simulink model "Model_2a_H2_batteries_primary_clean"  (R2019a)
settings: Solver=FixedStepAuto  StartTime=0.0  StopTime=8760  FixedStep=1  RelTol=1e-3
libraries: simulink x7
settings Model: Creator=senja  LastModifiedBy=senja

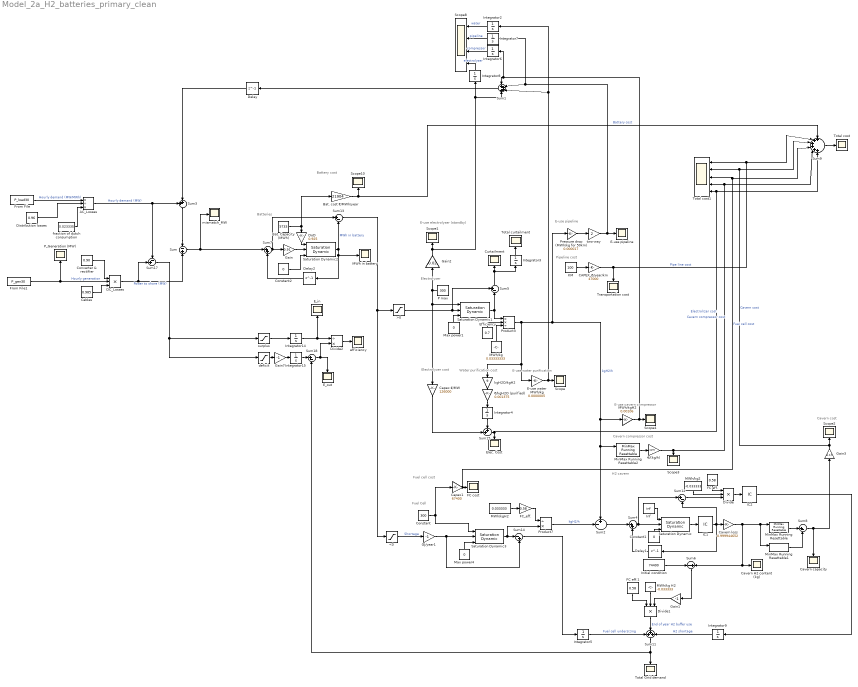
== system Model_2a_H2_batteries_primary_clean ==
  note: Water purification cost
  note: Batteries
  note: E-use pipeline
  note: E-use cavern compressor
  note: Cavern compressor cost
  note: Cavern cost
  note: E-use electrolyser (standby)
  note: E-use water purification
  note: Fuel cell cost
  note: Pipeline cost
  note: H2 cavern
  note: Fuel Cell
  note: Electrolyser
  note: Electrolyzer cost
  note: Battery cost
  <0 : Saturate  UpperLimit=0  LowerLimit=-inf
  >0 : Saturate  UpperLimit=inf  LowerLimit=-0
  AC_Losses : Product  Inputs=*/*
  Bat. Capacity (MWh) : Constant  Value=5733
  Bat. cost €/MWh/year : Gain  Gain=21904
  CAPEX_€/year/km : Gain  Gain=47000
  Cables : Constant  Value=0.985
  Capex €/MW : Gain  Gain=126000
  Capex1 : Gain  Gain=67400
  "Cavern H2 content (kg) " : Scope
  Cavern capacity : Scope
  Cavern loss : Gain  Gain=0.999944652
  Constant : Constant  Value=300
  Constant1 : Constant  Value=0
  Constant2 : Constant  Value=0
  Converter & rectifier : Constant  Value=0.90
  Curtailment : Scope
  DC_Losses : Product  Inputs=3
  Delay : Delay  DelayLength=1  InitialCondition=0
  Delay1 : Delay  DelayLength=1  InitialCondition=0
  Delay2 : Delay  DelayLength=1
  Distribution losses : Constant  Value=0.96
  Divide : Product  Inputs=***
  Divide1 : Product  Inputs=***
  Divide2 : Product  Inputs=/*
  DoD : Gain  Gain=0.925
  E-use pipeline : Scope
  E-use water MWh/kg : Gain  Gain=0.0000005
  E_in : Scope
  E_out : Scope
  Efficiency : Constant  Value=0.7
  Elec. Cost : Scope
  FC cost : Scope
  FC eff. : Constant  Value=0.58
  FC eff.1 : Constant  Value=0.58
  FC_eff. : Gain  Gain=0.58
  From File : FromFile  FileName=P_load30  SampleTime=0
  From File1 : FromFile  FileName=P_gen30  SampleTime=0
  GJ/year1 : Gain  Gain=-1
  Gain : Gain  Gain=0.91
  Gain1 : Gain  Gain=-1
  Gain2 : Gain  Gain=0.02
  Gain3 : Gain  Gain=0.17
  Gain7 : Gain  Gain=-1
  IC1 : InitialCondition  Value=74400
  IC2 : InitialCondition  Value=0
  Inf : Constant  Value=inf  OutDataTypeStr=Inherit: Inherit via back propagation
  Initial condition : Constant  Value=74400
  Integrator{2..9,14..15} (10 alike) : Integrator
  KM : Constant  Value=100
  "MWh in battery " : Scope
  MWh/kg : Constant  Value=0.03333333
  MWh/kg H2 : Constant  Value=-0.033333
  MWh/kg2 : Constant  Value=-0.033333
  MWh/kgH2 : Constant  Value=0.033333
  "MWh/kgH2 " : Gain  Gain=0.00106
  Max power1 : Constant  Value=0
  Max power4 : Constant  Value=0
  MinMax Running Resettable : simulink/Math Operations/MinMax Running Resettable  Function=max  vinit=0.0
  MinMax Running Resettable1 : simulink/Math Operations/MinMax Running Resettable  Function=min  vinit=0.0
  MinMax Running Resettable2 : simulink/Math Operations/MinMax Running Resettable  Function=max  vinit=0.0
  P max : Constant  Value=300
  P_Generation (MW) : Scope
  Pressure drop (MWh/kg for 50km) : Gain  Gain=0.000017
  Product3 : Product  Inputs=**/
  Product7 : Product  Inputs=/*
  Saturation Dynamic : simulink/Discontinuities/Saturation Dynamic  OutMin=0  OutMax=[]  OutDataTypeStr=Inherit: Same as second input  OutDataType=fixdt(1, 16)  OutScaling=2^-10  DoSatur=off
  Saturation Dynamic1 : simulink/Discontinuities/Saturation Dynamic  OutMin=[]  OutMax=[]  OutDataTypeStr=Inherit: Same as second input  OutDataType=fixdt(1, 16)  OutScaling=2^-10  DoSatur=off
  Saturation Dynamic2 : simulink/Discontinuities/Saturation Dynamic  OutMin=[]  OutMax=[]  OutDataTypeStr=Inherit: Same as second input  OutDataType=fixdt(1, 16)  OutScaling=2^-10  DoSatur=off
  Saturation Dynamic3 : simulink/Discontinuities/Saturation Dynamic  OutMin=[]  OutMax=[]  OutDataTypeStr=Inherit: Same as second input  OutDataType=fixdt(1, 16)  OutScaling=2^-10  DoSatur=off
  Scope{,1..4,10} (6 alike) : Scope
  Scope8 : Scope  NumInputPorts=4
  Sum : Sum  Inputs=-|+
  Sum1 : Sum  Inputs=++++
  Sum11 : Sum  Inputs=+++
  Sum{8,12..13,18} (4 alike) : Sum  Inputs=|+-
  Sum14 : Sum  Inputs=|-+
  Sum15 : Sum  Inputs=++|
  Sum17 : Sum  Inputs=-+|
  Sum2 : Sum  Inputs=+-|
  Sum3 : Sum  Inputs=++|
  Sum4 : Sum  Inputs=|++
  Sum5 : Sum  Inputs=+-|
  Sum6 : Sum  Inputs=-|+
  Sum7 : Sum  Inputs=|++
  Sum9 : Sum  Inputs=++++++
  Total Grid demand : Scope
  Total cost : Scope
  Total cost1 : Scope  NumInputPorts=5
  Total curtailment : Scope
  Transportation cost : Scope
  deficit : Saturate  UpperLimit=0  LowerLimit=-inf
  efficiency : Scope
  fraction of dutch consumption : Constant  Value=0.023335
  kgH2O/kgH2 : Gain  Gain=9
  mismatch_MW : Scope
  surplus : Saturate  UpperLimit=inf  LowerLimit=0
  two-way : Gain  Gain=2
  €/(kg/h) : Gain  Gain=1170
  €/kgH2O (purified) : Gain  Gain=0.001375
  wires:
  From File/1 -> AC_Losses/1  "Hourly demand (MW/MWh)"
  Efficiency/1 -> Product3/2
  fraction of dutch consumption/1 -> AC_Losses/3
  Distribution losses/1 -> AC_Losses/2
  Cables/1 -> DC_Losses/3
  Converter & rectifier/1 -> DC_Losses/1
  DC_Losses/1 -> Sum17/2, Sum/2  "Power to shore (MW)"
  >0/1 -> Sum5/1, Saturation Dynamic1/2
  <0/1 -> GJ/year1/1  "Shortage"
  AC_Losses/1 -> Sum3/1, Sum17/1  "Hourly demand (MW)"
  From File1/1 -> P_Generation (MW)/1, DC_Losses/2  "Hourly generation"
  Max power1/1 -> Saturation Dynamic1/3
  Saturation Dynamic1/1 -> Sum5/2, Product3/1
  Capex €/MW/1 -> Sum15/2
  Sum15/1 -> Elec. Cost/1, Sum9/6, Total cost1/5  "Electrolizer cost"
  €/kgH2O (purified)/1 -> Integrator4/1
  P max/1 -> Saturation Dynamic1/1, Capex €/MW/1, Gain2/1
  GJ/year1/1 -> Sum14/2, Saturation Dynamic3/2
  KM/1 -> CAPEX_€/year/km/1
  CAPEX_€/year/km/1 -> Total cost1/1, Sum9/2, Transportation cost/1  "Pipe line cost"
  Product3/1 -> E-use water MWh/kg/1, kgH2O/kgH2/1, "MWh/kgH2 "/1, MinMax Running Resettable2/1, Sum2/1, Pressure drop (MWh/kg for 50km)/1  "kgH2/h"
  Sum/1 -> Sum7/1, mismatch_MW/1
  Sum9/1 -> Total cost/1
  Constant/1 -> Saturation Dynamic3/1, Capex1/1
  Max power4/1 -> Saturation Dynamic3/3
  Saturation Dynamic3/1 -> Sum14/1, Product7/2
  MWh/kgH2/1 -> FC_eff./1
  Integrator3/1 -> Total curtailment/1
  kgH2O/kgH2/1 -> €/kgH2O (purified)/1
  Integrator4/1 -> Sum15/1
  MWh/kg/1 -> Product3/3
  Capex1/1 -> Total cost1/3, Sum9/4, FC cost/1  "Fuel cell cost"
  FC_eff./1 -> Product7/1
  Product7/1 -> Sum2/2  "kgH2/h"
  MinMax Running Resettable/1 -> Sum8/1
  MinMax Running Resettable1/1 -> Sum8/2
  Sum8/1 -> Cavern capacity/1, Gain3/1
  Sum5/1 -> Integrator3/1, Curtailment/1
  FC eff./1 -> Divide/1
  MWh/kg2/1 -> Divide/2
  Divide/1 -> IC2/1
  Sum14/1 -> Integrator5/1
  Initial condition/1 -> Sum6/1
  Integrator5/1 -> Sum11/1  "Fuel cell undersizing"
  Sum6/1 -> Gain1/1
  Sum11/1 -> Sum18/2, Total Grid demand/1
  Gain1/1 -> Divide1/3
  E-use water MWh/kg/1 -> Scope/1, Sum1/3, Integrator2/1
  Gain2/1 -> Scope1/1, Sum1/4, Integrator8/1
  Gain3/1 -> Sum9/3, Total cost1/2, Scope2/1  "Cavern cost"
  MinMax Running Resettable2/1 -> €/(kg/h)/1
  €/(kg/h)/1 -> Scope3/1, Sum9/5, Total cost1/4  "Cavern compressor cost"
  "MWh/kgH2 "/1 -> Sum1/1, Integrator6/1, Scope4/1
  Pressure drop (MWh/kg for 50km)/1 -> two-way/1
  two-way/1 -> E-use pipeline/1, Sum1/2, Integrator7/1
  Sum3/1 -> Sum/1
  Sum1/1 -> Delay/1
  Delay/1 -> Sum3/2
  MWh/kg H2/1 -> Divide1/2
  FC eff.1/1 -> Divide1/1
  Divide1/1 -> Sum11/2  "End of year H2 buffer use"
  Cavern loss/1 -> "Cavern H2 content (kg) "/1, Sum6/2, MinMax Running Resettable1/1, MinMax Running Resettable/1
  Sum12/1 -> Divide/3
  Delay1/1 -> Sum4/2
  Constant1/1 -> Saturation Dynamic/3
  Saturation Dynamic/1 -> IC1/1
  Sum4/1 -> Sum12/1, Saturation Dynamic/2
  IC1/1 -> Sum12/2, Cavern loss/1, Delay1/1
  Sum2/1 -> Sum4/1
  Inf/1 -> Saturation Dynamic/1
  IC2/1 -> Integrator9/1
  Integrator2/1 -> Scope8/1  "water"
  Integrator6/1 -> Scope8/3  "compressor"
  Integrator7/1 -> Scope8/2  "pipeline"
  Integrator8/1 -> Scope8/4  "electrolyser"
  Constant2/1 -> Saturation Dynamic2/3
  Sum7/1 -> Sum13/1, Gain/1
  Delay2/1 -> Sum7/2
  Sum13/1 -> <0/1, >0/1
  Bat. Capacity (MWh)/1 -> DoD/1, Bat. cost €/MWh/year/1
  Saturation Dynamic2/1 -> Delay2/1, "MWh in battery "/1, Sum13/2  "MWh in battery"
  Bat. cost €/MWh/year/1 -> Sum9/1, Scope10/1  "Battery cost"
  DoD/1 -> Saturation Dynamic2/1
  Gain/1 -> Saturation Dynamic2/2
  surplus/1 -> Integrator14/1
  Integrator14/1 -> E_in/1, Divide2/1
  deficit/1 -> Gain7/1
  Integrator15/1 -> Sum18/1
  Sum18/1 -> Divide2/2, E_out/1
  Gain7/1 -> Integrator15/1
  Sum17/1 -> surplus/1, deficit/1
  Divide2/1 -> efficiency/1
  Integrator9/1 -> Sum11/3  "H2 shortage"
